simulink model "Wind_Generation_Full_Group6_v2_R2019b"  (R2019b)
settings: Solver=ode23t  StartTime=0.0  StopTime=30  RelTol=1e-3
undefined symbols (not defined in the file): j
settings Model: Creator=pmout  LastModifiedBy=aspar

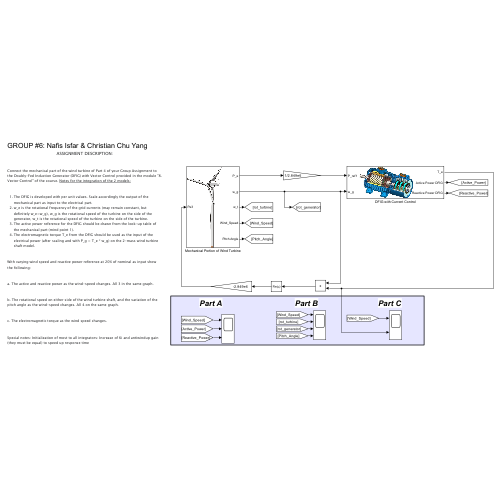
[thumbnail: Simulink's stored preview of the top-level diagram]
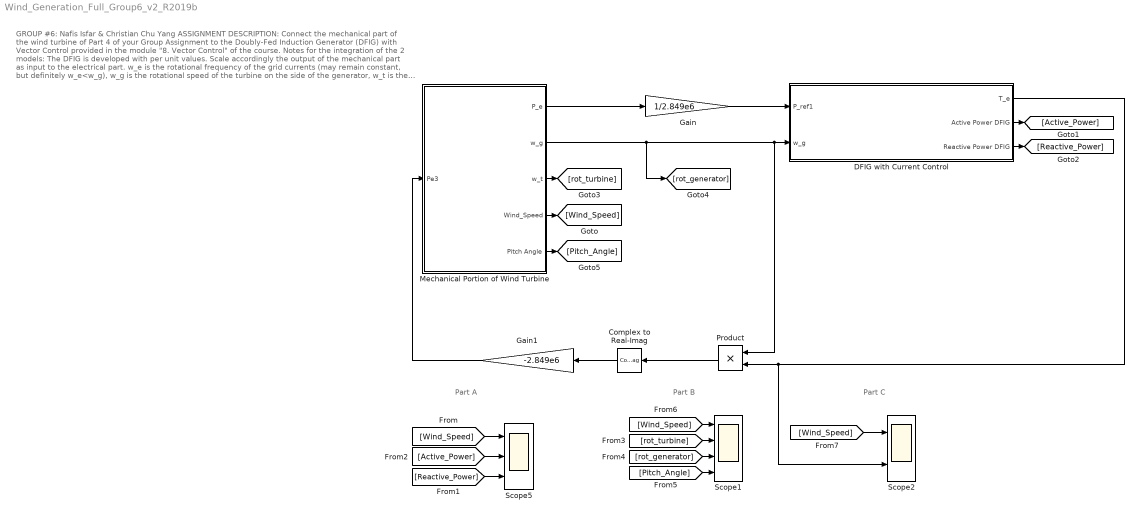
== system Wind_Generation_Full_Group6_v2_R2019b ==
  note: Part A
  note: GROUP #6: Nafis Isfar & Christian Chu Yang
      | ASSIGNMENT DESCRIPTION:
      | Connect the mechanical part of the wind turbine of Part 4 of your Group Assignment to the Doubly-Fed Induction Generator (DFIG) with Vector Control provided in the module "8. Vector Control" of the course. Notes for the integration of the 2 models:
      | The DFIG is developed with per unit values. Scale accordingly the output of the mechanical part as input to the electrical part.
      | w_e is the rotational frequency of the grid currents (may remain constant, but definitely w_e<w_g), w_g is the rotational speed of the turbine on the side of the generator, w_t is the rotational speed of the turbine on the side of the turbine.
      | The active power reference for the DFIG should be drawn from the look-up table of the mechanical part (mind point 1).
      | The electromagnetic torque T_e from the DFIG should be used as the input of the electrical power (after scaling and with P_g = T_e * w_g) on the 2-mass wind turbine shaft model.
      | With varying wind speed and reactive power reference at 20% of nominal as input show the following:
      | a. The active and reactive power as the wind-speed changes. All 3 in the same graph.
      | b. The rotational speed on either side of the wind turbine shaft, and the variation of the pitch angle as the wind-speed changes. All 4 on the same graph.
      | c. The electromagnetic torque as the wind speed changes.
      | Special notes: Initialization of most to all integrators: Increase of Ki and antiwindup gain (they must be equal) to speed up response time
  note: Part B
  note: Part C
  Complex to Real-Imag : ComplexToRealImag  Output=Real
  DFIG with Current Control : Subsystem  mask{Q_ref=0.2}
      mask prompts: Q_ref "Q_reference"
      mask Display: image('Doubly-fed-three-phase-induction-machine-with-rotary-transformer.png', [0,0,50,0,100,100]);
  Gain : Gain  Gain=1/2.849e6
  Gain1 : Gain  Gain=-2.849e6
  Mechanical Portion of Wind Turbine : Subsystem  mask{Parameter1=0}
      mask Display: image('wind_turbine.png', [0,0,50,0,100,100]);
  Product : Product
  Scope1 : Scope  NumInputPorts=4
  Scope2 : Scope  NumInputPorts=2
  Scope5 : Scope  NumInputPorts=3
  wires:
  Complex to Real-Imag/1 -> Gain1/1
  Product/1 -> Complex to Real-Imag/1
  Mechanical Portion of Wind Turbine/2(w_g) -> [rot_generator], Product/1, DFIG with Current Control/2(w_g)
  Gain1/1 -> Mechanical Portion of Wind Turbine/1(Pe3)
  Mechanical Portion of Wind Turbine/1(P_e) -> Gain/1
  Gain/1 -> DFIG with Current Control/1(P_ref1)
  DFIG with Current Control/1(T_e) -> Scope2/2, Product/2
  Mechanical Portion of Wind Turbine/4(Wind_Speed) -> [Wind_Speed]
  [Wind_Speed] -> Scope5/1
  DFIG with Current Control/2(Active Power DFIG) -> [Active_Power]
  DFIG with Current Control/3(Reactive Power DFIG) -> [Reactive_Power]
  [Active_Power] -> Scope5/2
  [Reactive_Power] -> Scope5/3
  Mechanical Portion of Wind Turbine/3(w_t) -> [rot_turbine]
  [Wind_Speed] -> Scope1/1
  [rot_generator] -> Scope1/3
  [rot_turbine] -> Scope1/2
  [Pitch_Angle] -> Scope1/4
  Mechanical Portion of Wind Turbine/5(Pitch Angle) -> [Pitch_Angle]
  [Wind_Speed] -> Scope2/1

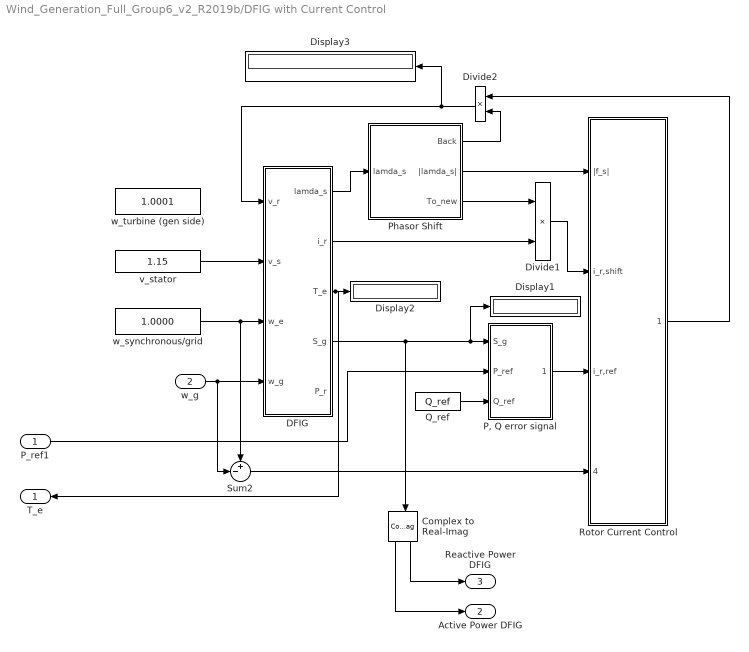
== system Wind_Generation_Full_Group6_v2_R2019b/DFIG with Current Control ==
  P_ref1 : Inport
  w_g : Inport  Port=2
  Complex to Real-Imag : ComplexToRealImag
  DFIG : Subsystem  mask{R_s=(4.6+4/100)*0.001, R_r=3.8e-3, L_m=1.99, L_s=(118.18+4/20)*0.001}
  Display1 : Display
  Display2 : Display
  Display3 : Display
  Divide1 : Product  Inputs=**
  Divide2 : Product  Inputs=**
  "P, Q error signal" : Subsystem  mask{p_err_ini=0.5555, q_err_ini=0.7527}
  Phasor Shift : Subsystem
  Q_ref : Constant  Value=Q_ref
  Rotor Current Control : Subsystem  mask{R_r=3.8e-3, L_s=(118.18+4/20)*0.001, t_ir=1.1, ini1=0.00286, ini2=0.00212}
      mask prompts: t_ir "ir control time constant"
  Sum2 : Sum  Inputs=+-|
  v_stator : Constant  Value=1.15
  w_synchronous/grid : Constant  Value=1.0000
  w_turbine (gen side) : Constant  Value=1.0001
  T_e : Outport
  Active Power DFIG : Outport  Port=2
  Reactive Power DFIG : Outport  Port=3
  wires:
  DFIG/4(S_g) -> Complex to Real-Imag/1, Display1/1, "P, Q error signal"/1(S_g)
  Q_ref/1 -> "P, Q error signal"/3(Q_ref)
  w_g/1 -> Sum2/2, DFIG/4(w_g)
  "P, Q error signal"/1(i_r,ref) -> Rotor Current Control/3(i_r,ref)
  Phasor Shift/2(|lamda_s|) -> Rotor Current Control/1(|f_s|)
  Divide2/1 -> Display3/1, DFIG/1(v_r)
  DFIG/3(T_e) -> T_e/1, Display2/1
  DFIG/1(lamda_s) -> Phasor Shift/1(lamda_s)
  Sum2/1 -> Rotor Current Control/4(w_e - w_g)
  v_stator/1 -> DFIG/2(v_s)
  Divide1/1 -> Rotor Current Control/2(i_r,shift)
  Rotor Current Control/1(v_r,shift) -> Divide2/1
  Phasor Shift/1(Back) -> Divide2/2
  w_synchronous/grid/1 -> DFIG/3(w_e), Sum2/1
  Phasor Shift/3(To_new) -> Divide1/1
  DFIG/2(i_r) -> Divide1/2
  P_ref1/1 -> "P, Q error signal"/2(P_ref)
  Complex to Real-Imag/2 -> Reactive Power DFIG/1
  Complex to Real-Imag/1 -> Active Power DFIG/1

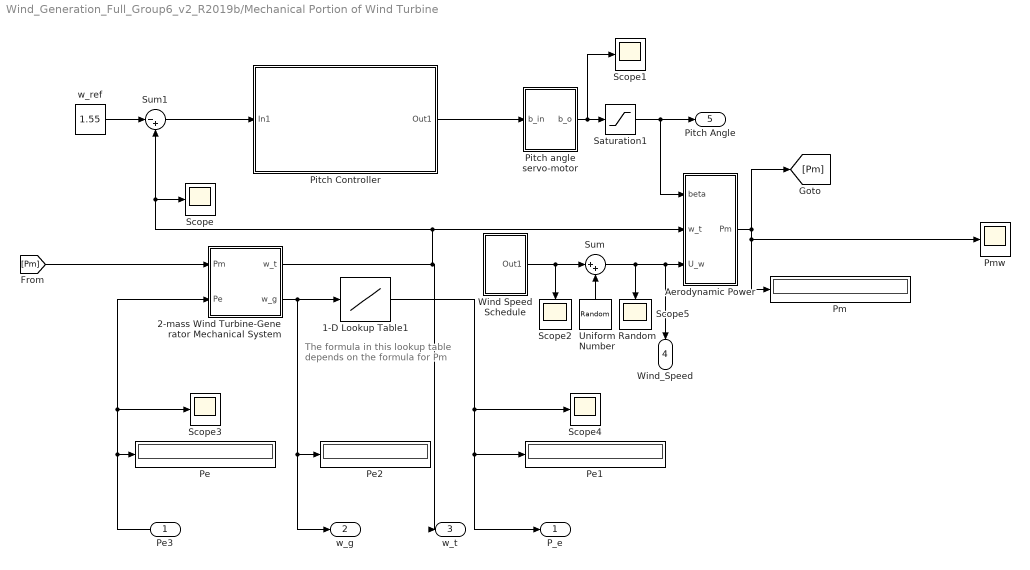
== system Wind_Generation_Full_Group6_v2_R2019b/Mechanical Portion of Wind Turbine ==
  note: The formula in this lookup table
      | depends on the formula for Pm
  Pe3 : Inport
  1-D Lookup Table1 : Lookup_n-D  NumberOfTableDimensions=1  BreakpointsForDimension1=[0:0.05:1.55]  Table=763e3*[0:0.05:1.55].^3 %648e3*[0:0.05:1.55].^3  InternalRulePriority=Speed  RndMeth=Simplest  InputSameDT=on
  2-mass Wind Turbine-Generator Mechanical System : Subsystem  mask{K=15e6, D=5e6, Jt=8e6, Jn=100, w_init=1.55, w_inig=1.55}
      mask prompts: K "Elasticity"; D "Damping"; Jt "Turb Moment of Inertia"; Jn "Gen Moment of Inertia"; w_init "Initial turb w"; w_inig "Initial gen w"
  Aerodynamic Power : Subsystem  mask{R=46, ro=1.225, z=[0.0095 0.033], c=[.26 116 .6  0 5 12.6]}
      mask prompts: R "Radius"; ro "Air density"; z "Z parameters"; c "C parameters"
  Pe : Display
  Pe1 : Display
  Pe2 : Display
  Pitch Controller : Subsystem  mask{init=1.55}
  Pitch angle servo-motor : Subsystem  mask{Tpam=0.2}
      mask prompts: Tpam "Pitch angle motor"
  Pm : Display
  Pmw : Scope
  Saturation1 : Saturate  UpperLimit=90  LowerLimit=0
  Scope{,1..5} (6 alike) : Scope
  Sum : Sum  Inputs=|++
  Sum1 : Sum  Inputs=|-+
  Uniform Random Number : UniformRandomNumber  Minimum=-0.3  Maximum=0.3  SampleTime=0.1
  Wind Speed Schedule : Subsystem
  w_ref : Constant  Value=1.55
  P_e : Outport
  w_g : Outport  Port=2
  w_t : Outport  Port=3
  Wind_Speed : Outport  Port=4
  Pitch Angle : Outport  Port=5
  wires:
  2-mass Wind Turbine-Generator Mechanical System/2(w_g) -> w_g/1, Pe2/1, 1-D Lookup Table1/1
  Saturation1/1 -> Pitch Angle/1, Aerodynamic Power/1(beta)
  Wind Speed Schedule/1(Out1) -> Scope2/1, Sum/1
  Pitch angle servo-motor/1(b_o) -> Scope1/1, Saturation1/1
  Aerodynamic Power/1(Pm) -> Pmw/1, Pm/1, [Pm]
  2-mass Wind Turbine-Generator Mechanical System/1(w_t) -> Aerodynamic Power/2(w_t), Scope/1, Sum1/2, w_t/1
  Sum1/1 -> Pitch Controller/1(In1)
  w_ref/1 -> Sum1/1
  Pe3/1 -> Scope3/1, 2-mass Wind Turbine-Generator Mechanical System/2(Pe), Pe/1
  Pitch Controller/1(Out1) -> Pitch angle servo-motor/1(b_in)
  1-D Lookup Table1/1 -> Scope4/1, P_e/1, Pe1/1
  [Pm] -> 2-mass Wind Turbine-Generator Mechanical System/1(Pm)
  Uniform Random Number/1 -> Sum/2
  Sum/1 -> Scope5/1, Wind_Speed/1, Aerodynamic Power/3(U_w)

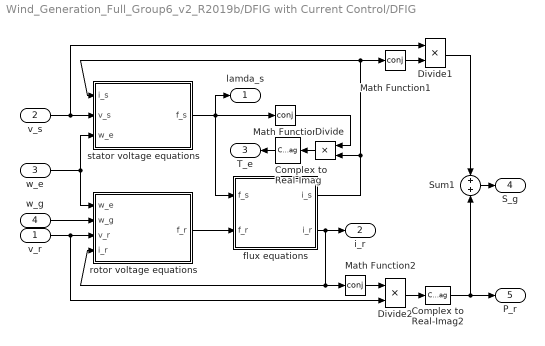
== system Wind_Generation_Full_Group6_v2_R2019b/DFIG with Current Control/DFIG ==
  v_r : Inport
  v_s : Inport  Port=2
  w_e : Inport  Port=3
  w_g : Inport  Port=4
  Complex to Real-Imag : ComplexToRealImag  Output=Imag
  Complex to Real-Imag2 : ComplexToRealImag  Output=Real
  Divide : Product  Inputs=**
  Divide1 : Product  Inputs=**
  Divide2 : Product  Inputs=**
  Math Function : Math  Operator=conj  SignedPower=on  SaturateOnIntegerOverflow=on
  Math Function1 : Math  Operator=conj  SignedPower=on  SaturateOnIntegerOverflow=on
  Math Function2 : Math  Operator=conj  SignedPower=on  SaturateOnIntegerOverflow=on
  Sum1 : Sum
  flux equations : Subsystem
  rotor voltage equations : Subsystem  mask{r_d_ini=-0.0002075, r_q_ini=0.003955}
  stator voltage equations : Subsystem  mask{s_d_ini=2.57e-06, s_q_ini=0.003671}
  lamda_s : Outport
  i_r : Outport  Port=2
  T_e : Outport  Port=3
  S_g : Outport  Port=4
  P_r : Outport  Port=5
  wires:
  Complex to Real-Imag2/1 -> P_r/1, Sum1/2
  Math Function2/1 -> Divide2/1
  stator voltage equations/1(f_s) -> flux equations/1(f_s), lamda_s/1, Math Function/1
  Math Function/1 -> Divide/1
  Divide2/1 -> Complex to Real-Imag2/1
  Divide1/1 -> Sum1/1
  Math Function1/1 -> Divide1/2
  Complex to Real-Imag/1 -> T_e/1
  Divide/1 -> Complex to Real-Imag/1
  rotor voltage equations/1(f_r) -> flux equations/2(f_r)
  flux equations/2(i_r) -> Math Function2/1, rotor voltage equations/4(i_r), i_r/1
  flux equations/1(i_s) -> Divide/2, stator voltage equations/1(i_s), Math Function1/1
  v_r/1 -> rotor voltage equations/3(v_r), Divide2/2
  w_e/1 -> rotor voltage equations/1(w_e), stator voltage equations/3(w_e)
  v_s/1 -> Divide1/1, stator voltage equations/2(v_s)
  w_g/1 -> rotor voltage equations/2(w_g)
  Sum1/1 -> S_g/1

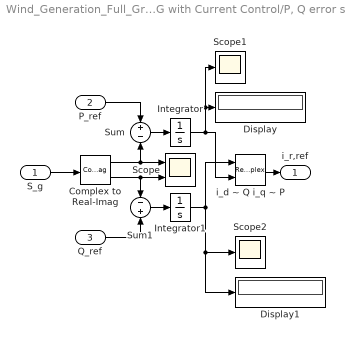
== system Wind_Generation_Full_Group6_v2_R2019b/DFIG with Current Control/P, Q error signal ==
  S_g : Inport
  P_ref : Inport  Port=2
  Q_ref : Inport  Port=3
  Complex to Real-Imag : ComplexToRealImag
  Display : Display
  Display1 : Display
  Integrator : Integrator  InitialCondition=p_err_ini
  Integrator1 : Integrator  InitialCondition=q_err_ini
  Scope : Scope  NumInputPorts=2
  Scope1 : Scope
  Scope2 : Scope
  Sum : Sum  Inputs=+|-
  Sum1 : Sum  Inputs=-|+
  i_d ~ Q i_q ~ P : RealImagToComplex
  i_r,ref : Outport
  wires:
  Sum/1 -> Integrator/1
  Complex to Real-Imag/2 -> Sum1/1, Scope/2
  i_d ~ Q i_q ~ P/1 -> i_r,ref/1
  Complex to Real-Imag/1 -> Sum/2, Scope/1
  Integrator/1 -> Scope1/1, Display/1, i_d ~ Q i_q ~ P/2
  Q_ref/1 -> Sum1/2
  Sum1/1 -> Integrator1/1
  Integrator1/1 -> Display1/1, Scope2/1, i_d ~ Q i_q ~ P/1
  P_ref/1 -> Sum/1
  S_g/1 -> Complex to Real-Imag/1

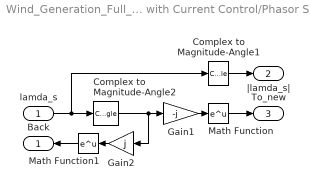
== system Wind_Generation_Full_Group6_v2_R2019b/DFIG with Current Control/Phasor Shift ==
  lamda_s : Inport
  Complex to Magnitude-Angle1 : ComplexToMagnitudeAngle  Output=Magnitude
  Complex to Magnitude-Angle2 : ComplexToMagnitudeAngle  Output=Angle
  Gain1 : Gain  Gain=-j
  Gain2 : Gain  Gain=j
  Math Function : Math  SignedPower=on  SaturateOnIntegerOverflow=on
  Math Function1 : Math  SignedPower=on  SaturateOnIntegerOverflow=on
  Back : Outport
  |lamda_s| : Outport  Port=2
  To_new : Outport  Port=3
  wires:
  Complex to Magnitude-Angle2/1 -> Gain2/1, Gain1/1
  Math Function1/1 -> Back/1
  Math Function/1 -> To_new/1
  Gain2/1 -> Math Function1/1
  Gain1/1 -> Math Function/1
  lamda_s/1 -> Complex to Magnitude-Angle1/1, Complex to Magnitude-Angle2/1
  Complex to Magnitude-Angle1/1 -> |lamda_s|/1

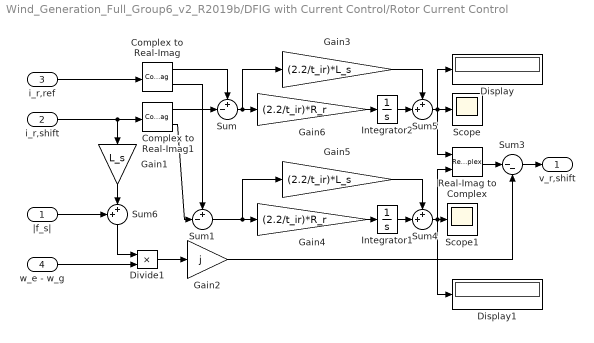
== system Wind_Generation_Full_Group6_v2_R2019b/DFIG with Current Control/Rotor Current Control ==
  |f_s| : Inport
  i_r,shift : Inport  Port=2
  i_r,ref : Inport  Port=3
  w_e - w_g : Inport  Port=4
  Complex to Real-Imag : ComplexToRealImag
  Complex to Real-Imag1 : ComplexToRealImag
  Display : Display
  Display1 : Display
  Divide1 : Product  Inputs=**
  Gain1 : Gain  Gain=L_s
  Gain2 : Gain  Gain=j
  Gain3 : Gain  Gain=(2.2/t_ir)*L_s
  Gain4 : Gain  Gain=(2.2/t_ir)*R_r
  Gain5 : Gain  Gain=(2.2/t_ir)*L_s
  Gain6 : Gain  Gain=(2.2/t_ir)*R_r
  Integrator1 : Integrator  InitialCondition=ini2
  Integrator2 : Integrator  InitialCondition=ini1
  Real-Imag to Complex : RealImagToComplex
  Scope : Scope
  Scope1 : Scope
  Sum : Sum  Inputs=+-|
  Sum1 : Sum  Inputs=+-|
  Sum3 : Sum  Inputs=|--
  Sum4 : Sum  Inputs=++|
  Sum5 : Sum  Inputs=++|
  Sum6 : Sum  Inputs=++|
  v_r,shift : Outport
  wires:
  Gain2/1 -> Sum3/2
  Sum6/1 -> Divide1/1
  Gain1/1 -> Sum6/2
  |f_s|/1 -> Sum6/1
  Gain3/1 -> Sum5/1
  Gain5/1 -> Sum4/1
  Sum4/1 -> Display1/1, Scope1/1, Real-Imag to Complex/2
  Sum5/1 -> Display/1, Scope/1, Real-Imag to Complex/1
  Gain6/1 -> Integrator2/1
  Integrator2/1 -> Sum5/2
  Sum1/1 -> Gain4/1, Gain5/1
  Gain4/1 -> Integrator1/1
  Integrator1/1 -> Sum4/2
  Divide1/1 -> Gain2/1
  Sum3/1 -> v_r,shift/1
  Real-Imag to Complex/1 -> Sum3/1
  w_e - w_g/1 -> Divide1/2
  Complex to Real-Imag1/2 -> Sum1/2
  Complex to Real-Imag1/1 -> Sum/2
  i_r,shift/1 -> Gain1/1, Complex to Real-Imag1/1
  Complex to Real-Imag/2 -> Sum1/1
  Complex to Real-Imag/1 -> Sum/1
  i_r,ref/1 -> Complex to Real-Imag/1
  Sum/1 -> Gain3/1, Gain6/1

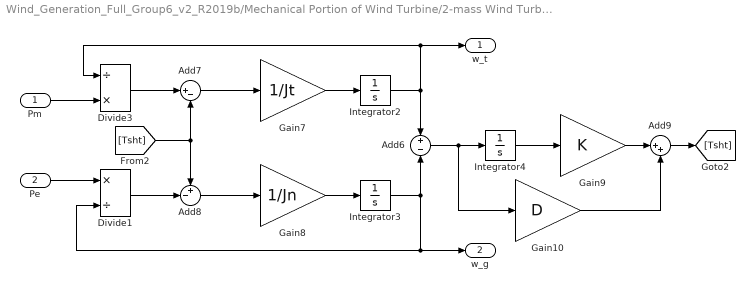
== system Wind_Generation_Full_Group6_v2_R2019b/Mechanical Portion of Wind Turbine/2-mass Wind Turbine-Generator Mechanical System ==
  Pm : Inport
  Pe : Inport  Port=2
  Add6 : Sum  Inputs=+|-
  Add7 : Sum  Inputs=|+-
  Add8 : Sum  Inputs=+-|
  Add9 : Sum  Inputs=|++
  Divide1 : Product  Inputs=*/
  Divide3 : Product  Inputs=/*
  Gain10 : Gain  Gain=D
  Gain7 : Gain  Gain=1/Jt
  Gain8 : Gain  Gain=1/Jn
  Gain9 : Gain  Gain=K
  Integrator2 : Integrator  InitialCondition=w_init
  Integrator3 : Integrator  InitialCondition=w_inig
  Integrator4 : Integrator  InitialCondition=0.35
  w_t : Outport
  w_g : Outport  Port=2
  wires:
  Add9/1 -> [Tsht]
  Gain8/1 -> Integrator3/1
  Integrator2/1 -> Add6/1, Divide3/1, w_t/1
  Gain7/1 -> Integrator2/1
  Add6/1 -> Gain10/1, Integrator4/1
  Integrator3/1 -> Divide1/2, w_g/1, Add6/2
  Integrator4/1 -> Gain9/1
  Divide1/1 -> Add8/2
  Gain10/1 -> Add9/2
  [Tsht] -> Add8/1, Add7/2
  Divide3/1 -> Add7/1
  Gain9/1 -> Add9/1
  Add8/1 -> Gain8/1
  Add7/1 -> Gain7/1
  Pe/1 -> Divide1/1
  Pm/1 -> Divide3/2

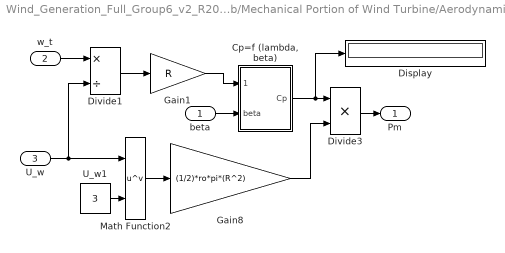
== system Wind_Generation_Full_Group6_v2_R2019b/Mechanical Portion of Wind Turbine/Aerodynamic Power ==
  beta : Inport
  w_t : Inport  Port=2
  U_w : Inport  Port=3
  "Cp=f (lambda, beta)" : Subsystem
  Display : Display
  Divide1 : Product  Inputs=*/
  Divide3 : Product  Inputs=**
  Gain1 : Gain  Gain=R
  Gain8 : Gain  Gain=(1/2)*ro*pi*(R^2)
  Math Function2 : Math  Operator=pow  SaturateOnIntegerOverflow=on
  U_w1 : Constant  Value=3
  Pm : Outport
  wires:
  U_w/1 -> Divide1/2, Math Function2/1
  Math Function2/1 -> Gain8/1
  Divide3/1 -> Pm/1
  U_w1/1 -> Math Function2/2
  Gain8/1 -> Divide3/2
  "Cp=f (lambda, beta)"/1(Cp) -> Display/1, Divide3/1
  beta/1 -> "Cp=f (lambda, beta)"/2(beta)
  w_t/1 -> Divide1/1
  Divide1/1 -> Gain1/1
  Gain1/1 -> "Cp=f (lambda, beta)"/1(lambda)

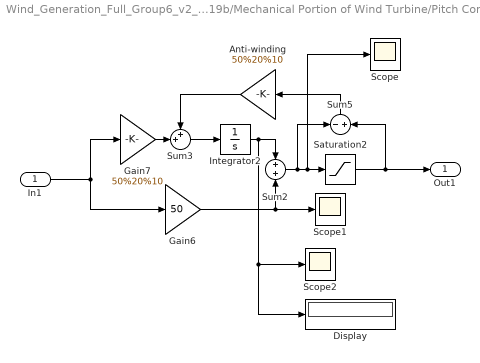
== system Wind_Generation_Full_Group6_v2_R2019b/Mechanical Portion of Wind Turbine/Pitch Controller ==
  In1 : Inport
  Anti-winding : Gain  Gain=50%20%10
  Display : Display
  Gain6 : Gain  Gain=50
  Gain7 : Gain  Gain=50%20%10
  Integrator2 : Integrator  InitialCondition=0.34
  Saturation2 : Saturate  UpperLimit=90  LowerLimit=0
  Scope : Scope
  Scope1 : Scope
  Scope2 : Scope
  Sum2 : Sum  Inputs=+|+
  Sum3 : Sum  Inputs=++|
  Sum5 : Sum  Inputs=-|+
  Out1 : Outport
  wires:
  Integrator2/1 -> Sum2/1, Display/1, Scope2/1
  Sum5/1 -> Anti-winding/1
  Gain7/1 -> Sum3/2
  Sum2/1 -> Sum5/1, Scope/1, Saturation2/1
  Sum3/1 -> Integrator2/1
  Anti-winding/1 -> Sum3/1
  Gain6/1 -> Scope1/1, Sum2/2
  In1/1 -> Gain7/1, Gain6/1
  Saturation2/1 -> Out1/1, Sum5/2

== system Wind_Generation_Full_Group6_v2_R2019b/Mechanical Portion of Wind Turbine/Pitch angle servo-motor ==
  b_in : Inport
  Display : Display
  Gain8 : Gain  Gain=1/Tpam
  Integrator3 : Integrator
  Saturation2 : Saturate  UpperLimit=8  LowerLimit=-8
  Scope : Scope
  Sum3 : Sum  Inputs=|+-
  b_o : Outport
  wires:
  Sum3/1 -> Gain8/1
  b_in/1 -> Sum3/1
  Gain8/1 -> Saturation2/1
  Integrator3/1 -> Sum3/2, Display/1, Scope/1, b_o/1
  Saturation2/1 -> Integrator3/1

== system Wind_Generation_Full_Group6_v2_R2019b/Mechanical Portion of Wind Turbine/Wind Speed Schedule ==
  Add : Sum  Inputs=+++++
  Scope : Scope
  Step : Step  Time=5  Before=11.1  After=8  SampleTime=0
  Step1 : Step  Time=10  After=4  SampleTime=0
  Step2 : Step  Time=15  After=4  SampleTime=0
  Step3 : Step  Time=20  After=2  SampleTime=0
  Step4 : Step  Time=25  After=-8  SampleTime=0
  U_w : Constant  Value=11.1
  Out1 : Outport
  wires:
  Add/1 -> Scope/1, Out1/1
  Step4/1 -> Add/5
  Step3/1 -> Add/4
  Step2/1 -> Add/3
  Step1/1 -> Add/2
  Step/1 -> Add/1

== system Wind_Generation_Full_Group6_v2_R2019b/DFIG with Current Control/DFIG/flux equations ==
  f_s : Inport
  f_r : Inport  Port=2
  Gain5 : Gain  Gain=1/L_s
  Gain7 : Gain  Gain=1/L_m
  Sum1 : Sum  Inputs=|+-
  Sum5 : Sum  Inputs=-+|
  i_s : Outport
  i_r : Outport  Port=2
  wires:
  Sum1/1 -> i_s/1
  Gain7/1 -> Sum1/1
  Sum5/1 -> Gain5/1
  f_r/1 -> Sum5/2
  Gain5/1 -> Sum1/2, i_r/1
  f_s/1 -> Sum5/1, Gain7/1

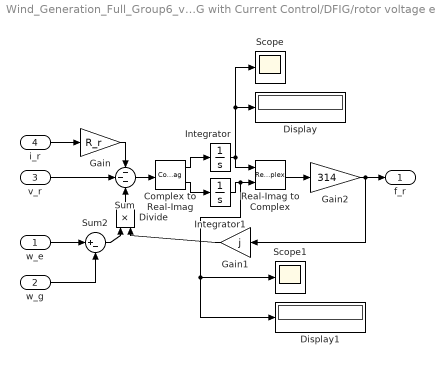
== system Wind_Generation_Full_Group6_v2_R2019b/DFIG with Current Control/DFIG/rotor voltage equations ==
  w_e : Inport
  w_g : Inport  Port=2
  v_r : Inport  Port=3
  i_r : Inport  Port=4
  Complex to Real-Imag : ComplexToRealImag
  Display : Display
  Display1 : Display
  Divide : Product  Inputs=**
  Gain : Gain  Gain=R_r
  Gain1 : Gain  Gain=j
  Gain2 : Gain  Gain=314
  Integrator : Integrator  InitialCondition=r_d_ini
  Integrator1 : Integrator  InitialCondition=r_q_ini
  Real-Imag to Complex : RealImagToComplex
  Scope : Scope
  Scope1 : Scope
  Sum : Sum  Inputs=---
  Sum2 : Sum  Inputs=|+-
  f_r : Outport
  wires:
  Gain2/1 -> Gain1/1, f_r/1
  Gain1/1 -> Divide/2
  Complex to Real-Imag/2 -> Integrator1/1
  Complex to Real-Imag/1 -> Integrator/1
  Sum/1 -> Complex to Real-Imag/1
  w_g/1 -> Sum2/2
  w_e/1 -> Sum2/1
  Gain/1 -> Sum/1
  v_r/1 -> Sum/2
  i_r/1 -> Gain/1
  Real-Imag to Complex/1 -> Gain2/1
  Sum2/1 -> Divide/1
  Divide/1 -> Sum/3
  Integrator1/1 -> Display1/1, Scope1/1, Real-Imag to Complex/2
  Integrator/1 -> Display/1, Scope/1, Real-Imag to Complex/1

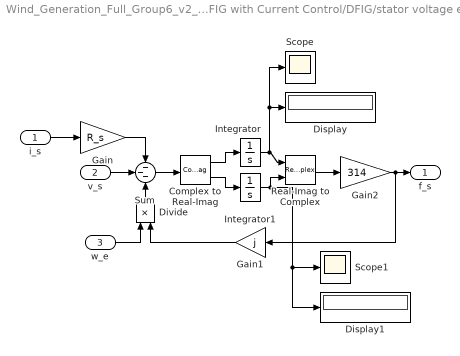
== system Wind_Generation_Full_Group6_v2_R2019b/DFIG with Current Control/DFIG/stator voltage equations ==
  i_s : Inport
  v_s : Inport  Port=2
  w_e : Inport  Port=3
  Complex to Real-Imag : ComplexToRealImag
  Display : Display
  Display1 : Display
  Divide : Product  Inputs=**
  Gain : Gain  Gain=R_s
  Gain1 : Gain  Gain=j
  Gain2 : Gain  Gain=314
  Integrator : Integrator  InitialCondition=s_d_ini
  Integrator1 : Integrator  InitialCondition=s_q_ini
  Real-Imag to Complex : RealImagToComplex
  Scope : Scope
  Scope1 : Scope
  Sum : Sum  Inputs=---
  f_s : Outport
  wires:
  Gain2/1 -> Gain1/1, f_s/1
  Gain1/1 -> Divide/2
  Complex to Real-Imag/2 -> Integrator1/1
  Complex to Real-Imag/1 -> Integrator/1
  Sum/1 -> Complex to Real-Imag/1
  v_s/1 -> Sum/2
  Gain/1 -> Sum/1
  i_s/1 -> Gain/1
  Real-Imag to Complex/1 -> Gain2/1
  w_e/1 -> Divide/1
  Divide/1 -> Sum/3
  Integrator1/1 -> Display1/1, Scope1/1, Real-Imag to Complex/2
  Integrator/1 -> Scope/1, Display/1, Real-Imag to Complex/1

== system Wind_Generation_Full_Group6_v2_R2019b/Mechanical Portion of Wind Turbine/Aerodynamic Power/Cp=f (lambda, beta) ==
  lambda : Inport
  beta : Inport  Port=2
  Cp=f (lambda,beta,li) : Fcn  Expr=c(1)*(c(2)*u(3)-c(3)*u(2)-c(4)*(u(2)^1)-c(5) )*exp(-c(6)*u(3))  SampleTime=0
  Mux : Mux  Inputs=2
  Mux1 : Mux  Inputs=2
  li=f(lambda,beta) : Fcn  Expr=1/(u(1)+z(1)*u(2))-z(2)/(u(2)^3+1)  SampleTime=0
  Cp : Outport
  wires:
  Cp=f (lambda,beta,li)/1 -> Cp/1
  beta/1 -> Mux/2
  lambda/1 -> Mux/1
  li=f(lambda,beta)/1 -> Mux1/2
  Mux1/1 -> Cp=f (lambda,beta,li)/1
  Mux/1 -> Mux1/1, li=f(lambda,beta)/1
